simulink model "Ann_EMG"  (Simulink 6.6)
settings: Solver=ode45  StartTime=0.0  StopTime=inf  RelTol=1e-3
undefined symbols (not defined in the file or in its folder): analoginput
libraries: daqlib x1
settings Model: Creator=cmcrae  LastModifiedBy=training

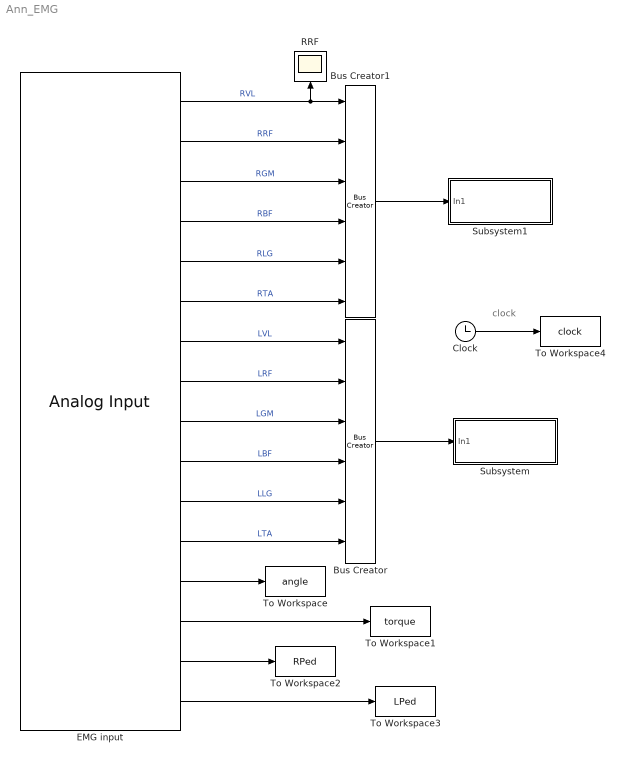
== system Ann_EMG ==
  note: clock
  Bus Creator : BusCreator  Inputs=6
  Bus Creator1 : BusCreator  Inputs=6
  Clock : Clock
      settings: Decimation=10
  EMG input : daqlib/Analog Input  DialogController=daqcreatedialog  DialogControllerArgs=DataTag0  AcqMode=0  Device=nidaq Dev1 (USB-6210)  ObjConstructor=analoginput('nidaq','Dev1')  SampleRate=4000  ActualRate=4000  SamplesPerFrame=2  InputType=SingleEnded  NChannelsSelected=16  Channels=1$0$$1$#1$1$$1$#1$2$$1$#1$3$$1$#1$4$$1$#1$5$$1$#1$6$$1$#1$7$$1$#1$8$$1$#1$9$$1$#1$10$$1$#1$11$$1$#1$12$$1$#1$13$$1$#1$14$$1$#1$15$$1$#  NPorts=1 per hardware channel  DataType=double
      settings: SignalType=Sample-based
  RRF : Scope
      settings: Orientation=up  YMin=-0.175  YMax=0.15  SaveName=ScopeData2
  Subsystem : Subsystem
  Subsystem1 : Subsystem
  To Workspace : ToWorkspace  VariableName=angle  SampleTime=-1  SaveFormat=Structure
  To Workspace1 : ToWorkspace  VariableName=torque  SampleTime=-1  SaveFormat=Structure
  To Workspace2 : ToWorkspace  VariableName=RPed  SampleTime=-1  SaveFormat=Structure
  To Workspace3 : ToWorkspace  VariableName=LPed  SampleTime=-1  SaveFormat=Structure
  To Workspace4 : ToWorkspace  VariableName=clock  SampleTime=-1  SaveFormat=Structure
  wires:
  EMG input/7 -> Bus Creator/1  "LVL"
  EMG input/1 -> Bus Creator1/1, RRF/1  "RVL"
  EMG input/2 -> Bus Creator1/2  "RRF"
  EMG input/3 -> Bus Creator1/3  "RGM"
  EMG input/4 -> Bus Creator1/4  "RBF"
  EMG input/5 -> Bus Creator1/5  "RLG"
  EMG input/6 -> Bus Creator1/6  "RTA"
  Bus Creator1/1 -> Subsystem1/1(In1)
  EMG input/8 -> Bus Creator/2  "LRF"
  EMG input/9 -> Bus Creator/3  "LGM"
  EMG input/10 -> Bus Creator/4  "LBF"
  EMG input/11 -> Bus Creator/5  "LLG"
  EMG input/12 -> Bus Creator/6  "LTA"
  Bus Creator/1 -> Subsystem/1(In1)
  EMG input/13 -> To Workspace/1
  EMG input/14 -> To Workspace1/1
  EMG input/15 -> To Workspace2/1
  EMG input/16 -> To Workspace3/1
  Clock/1 -> To Workspace4/1

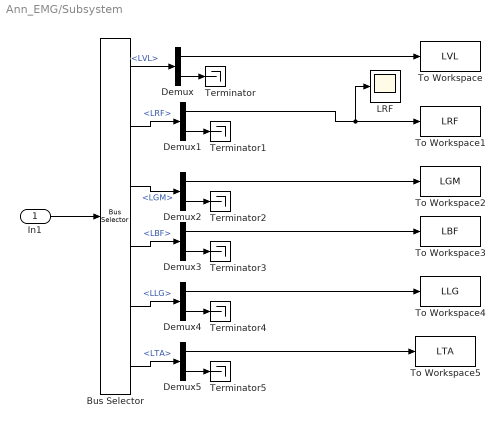
== system Ann_EMG/Subsystem ==
  In1 : Inport
  Bus Selector : BusSelector  OutputSignals=LVL,LRF,LGM,LBF,LLG,LTA
  Demux{,1..5} (6 alike) : Demux  Outputs=2
  LRF : Scope
  Terminator{,1..5} (6 alike) : Terminator
  To Workspace : ToWorkspace  VariableName=LVL  SampleTime=-1  SaveFormat=Structure
  To Workspace1 : ToWorkspace  VariableName=LRF  SampleTime=-1  SaveFormat=Structure
  To Workspace2 : ToWorkspace  VariableName=LGM  SampleTime=-1  SaveFormat=Structure
  To Workspace3 : ToWorkspace  VariableName=LBF  SampleTime=-1  SaveFormat=Structure
  To Workspace4 : ToWorkspace  VariableName=LLG  SampleTime=-1  SaveFormat=Structure
  To Workspace5 : ToWorkspace  VariableName=LTA  SampleTime=-1  SaveFormat=Structure
  wires:
  In1/1 -> Bus Selector/1
  Bus Selector/1 -> Demux/1  "<LVL>"
  Demux/2 -> Terminator/1
  Demux/1 -> To Workspace/1
  Demux1/2 -> Terminator1/1
  Demux2/2 -> Terminator2/1
  Demux2/1 -> To Workspace2/1
  Demux3/2 -> Terminator3/1
  Demux4/2 -> Terminator4/1
  Demux5/2 -> Terminator5/1
  Bus Selector/2 -> Demux1/1  "<LRF>"
  Bus Selector/3 -> Demux2/1  "<LGM>"
  Bus Selector/4 -> Demux3/1  "<LBF>"
  Bus Selector/5 -> Demux4/1  "<LLG>"
  Bus Selector/6 -> Demux5/1  "<LTA>"
  Demux1/1 -> To Workspace1/1, LRF/1
  Demux3/1 -> To Workspace3/1
  Demux4/1 -> To Workspace4/1
  Demux5/1 -> To Workspace5/1

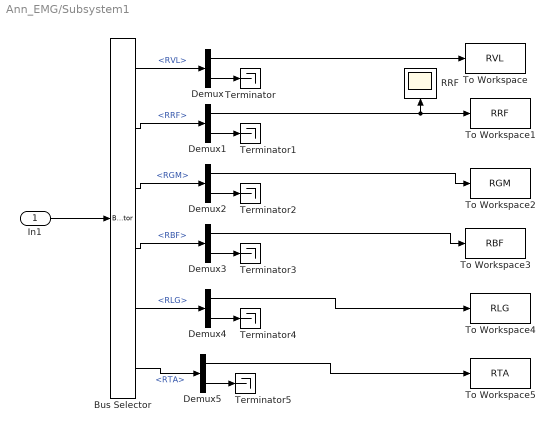
== system Ann_EMG/Subsystem1 ==
  In1 : Inport
  Bus Selector : BusSelector  OutputSignals=RVL,RRF,RGM,RBF,RLG,RTA
  Demux{,1..5} (6 alike) : Demux  Outputs=2
  RRF : Scope
      settings: Orientation=up
  Terminator{,1..5} (6 alike) : Terminator
  To Workspace : ToWorkspace  VariableName=RVL  SampleTime=-1  SaveFormat=Structure
  To Workspace1 : ToWorkspace  VariableName=RRF  SampleTime=-1  SaveFormat=Structure
  To Workspace2 : ToWorkspace  VariableName=RGM  SampleTime=-1  SaveFormat=Structure
  To Workspace3 : ToWorkspace  VariableName=RBF  SampleTime=-1  SaveFormat=Structure
  To Workspace4 : ToWorkspace  VariableName=RLG  SampleTime=-1  SaveFormat=Structure
  To Workspace5 : ToWorkspace  VariableName=RTA  SampleTime=-1  SaveFormat=Structure
  wires:
  In1/1 -> Bus Selector/1
  Bus Selector/1 -> Demux/1  "<RVL>"
  Demux/1 -> To Workspace/1
  Demux/2 -> Terminator/1
  Bus Selector/2 -> Demux1/1  "<RRF>"
  Demux1/2 -> Terminator1/1
  Demux1/1 -> To Workspace1/1, RRF/1
  Bus Selector/3 -> Demux2/1  "<RGM>"
  Demux2/2 -> Terminator2/1
  Demux2/1 -> To Workspace2/1
  Bus Selector/4 -> Demux3/1  "<RBF>"
  Demux3/2 -> Terminator3/1
  Demux3/1 -> To Workspace3/1
  Demux4/2 -> Terminator4/1
  Bus Selector/5 -> Demux4/1  "<RLG>"
  Demux4/1 -> To Workspace4/1
  Demux5/2 -> Terminator5/1
  Demux5/1 -> To Workspace5/1
  Bus Selector/6 -> Demux5/1  "<RTA>"
